simulink library "Quaternion_Conjugate"  (R2016a)
settings: Solver=ode45  StartTime=0.0  StopTime=10.0  RelTol=1e-3
settings Model: Creator=devantormey  LastModifiedBy=devantormey
settings DataIOCC: LimitDataPoints=on
settings DebuggingCC: AllowSymbolicDim=off

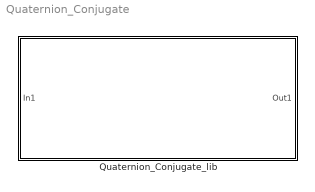
== system Quaternion_Conjugate ==
  Quaternion_Conjugate_lib : Subsystem

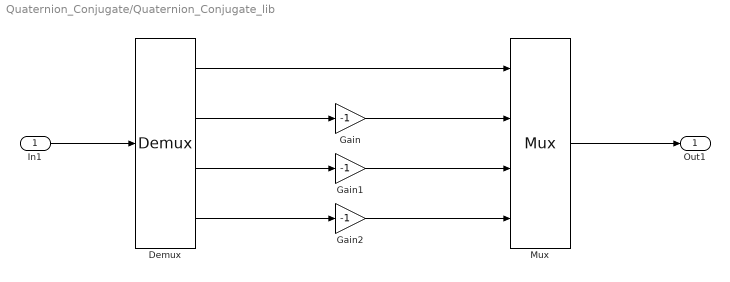
== system Quaternion_Conjugate/Quaternion_Conjugate_lib ==
  In1 : Inport
  Demux : Demux
  Gain : Gain  Gain=-1
  Gain1 : Gain  Gain=-1
  Gain2 : Gain  Gain=-1
  Mux : Mux
  Out1 : Outport
  wires:
  In1/1 -> Demux/1
  Demux/1 -> Mux/1
  Demux/2 -> Gain/1
  Gain/1 -> Mux/2
  Demux/3 -> Gain1/1
  Gain1/1 -> Mux/3
  Demux/4 -> Gain2/1
  Gain2/1 -> Mux/4
  Mux/1 -> Out1/1
